simulink model "MQP_RHOME_2025"  (R2024b)
settings: Solver=VariableStepAuto  StartTime=0.0  StopTime=24  RelTol=1e-3  EnableMultiTasking=on
undefined symbols (not defined in the file): DiscIntNeverNeededParam, Ion, Lithium
libraries: spsSeriesRLCBranchLib x11, simulink x11, powerlib_extras x11, spsVoltageMeasurementLib x10, spsGroundLib x4, dspmathops x3, spsUniversalBridgeLib x3, spsMeanLib x3, slpidlib x3, spsCurrentMeasurementLib x2, spsMosfetLib x2, spsThreePhaseParallelRLCBranchLib x2
(part 1 of 3)
settings Model: SimulationMode=accelerator  Creator=yaju  LastModifiedBy=thomasrua
settings SolverCC: AlgebraicLoopSolver=TrustRegion
settings DataIOCC: ReturnWorkspaceOutputs=off
settings OptimizationCC: LifeSpan=inf
settings DebuggingCC: UnconnectedInputMsg=warning  UnconnectedOutputMsg=warning  UnconnectedLineMsg=warning  SFUnexpectedBacktrackingDiag=warning  SFNoUnconditionalDefaultTransitionDiag=warning  SFExecutionAtInitializationDiag=none  ArithmeticOperatorsInVariantConditions=warning
settings ModelReferenceCC: EnableRefExpFcnMdlSchedulingChecks=on
settings SFSimCC: SimUseLocalCustomCode=off  CustomCodeUndefinedFunction=UseInterfaceOnly
settings RTWCC: RTWUseLocalCustomCode=off  GPUComputeCapability=3.5
settings CodeAppCC: StateflowObjectComments=on
settings GRTTargetCC: TargetLangStandard=C89/C90 (ANSI)
settings ConfigComp: CovMetricSettings=dw  CovSaveCumulativeToWorkspaceVar=on  CovSaveSingleToWorkspaceVar=on  CovExternalEMLEnable=off
settings SimscapeCC: SimscapeNormalizeSystem=off

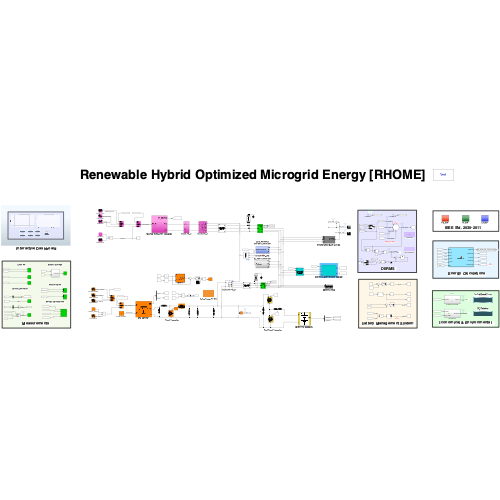
[thumbnail: Simulink's stored preview of the top-level diagram]
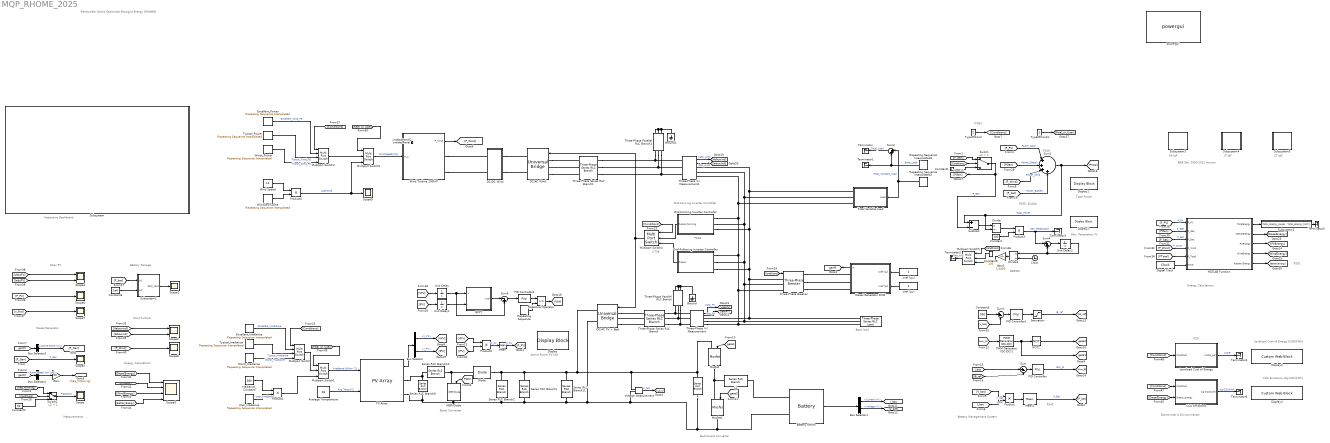
== system MQP_RHOME_2025 ==
  note: Levelized Cost of Energy
      | [USD/kWh]
  note: IT20
  note: PS48
  note: PS49
  note: PS51
  note: PS55: SCADA
  note: PS42
  note: CT39
  note: ITN01
  note: IEEE Std. 2030-2011 Axioms
  note: Economical & Environmental
  note: Grid-Forming
      | Inverter Controller
  note: Measurements
  note: DERMS
  note: Base load
  note: Battery Management System
  note: Buck/boost Converter
  note: Renewable Hybrid Optimized Microgrid Energy [RHOME]
  note: Active Power PV [W]
  note: Interactive Dashboard
  note: Boost Converter
  note: Energy Calculations
  note: Total Power
  note: Ren. Penetration %
  note: Diesel Generator
  note: Solar PV
  note: Battery Storage
  note: Wind Turbine
  note: Energy Calculations
  note: PS-IAP
  note: CT-IAP
  note: IT-IAP
  note: CO2 Emissions
      | [Kg-CO2/kWh]
  " " : spsThreePhaseSeriesRLCLoadLib/Three-Phase Series RLC Load  LConnTagsString=A|B|C  Configuration=Y (grounded)  NominalVoltage=400  Vabc=[1e3 1e3 1e3]  Vabcp=[1e3 1e3 1e3]  NominalFrequency=50  UnbalancedPower=off  ActivePower=83e3  InductivePower=5e3  CapacitivePower=5e3  Pabc=[10e3 9e3 11e3]  QLabc=[100 90 110]  QCabc=[100 90 110]  Pabcp=[10e3 9e3 11e3]  QLabcp=[100 90 110]  QCabcp=[100 90 110]  Measurements=Branch voltages and currents  LoadType=constant PQ
  "      R" : spsSeriesRLCBranchLib/Series RLC Branch  LConnTagsString=__new0  RConnTagsString=__new0  BranchType=RC  Resistance=1e-4  Inductance=1000e-6  SetiL0=off  InitialCurrent=0  Capacitance=210e-6  Setx0=off  InitialVoltage=0  Measurements=None
  "Average Temperature " : Constant  Value=28
  "Battery 6MWh " : spsBatteryLib/Battery  BatType=Lithium-Ion  NomV=230  NomQ=26087  SOC=50  Batt_Tr=1  PresetModel=on  MaxQ=26087  MinV=172.5  FullV=267.717  Dis_rate=11342.1739  R=8.8167e-05  Normal_OP=23591.7217  expZone="[248.48875      1281.6657]"
      settings: LibrarySourceBlock=electricdrivelib/Extra Sources/Battery
  Bus Selector : BusSelector  OutputSignals=V_PV,I_PV
  Bus Selector1 : BusSelector  OutputSignals=Current (A),Voltage (V)
  Bus Selector3 : BusSelector  OutputSignals=Active Power (W)
  Bus Selector4 : BusSelector  OutputSignals="Rotor speed  wm  (pu)"
  CO2 Emissions : Subsystem
  Clock : Clock
  Constant : Constant  Value=100
  Constant1 : Constant  Value=0
  Constant2 : Constant  Value=50
  Constant3 : Constant  Value=550
  Constant4 : Constant  Value=1e6
  Constant5 : Constant  Value=100
  DC/AC PV + Batt : spsUniversalBridgeLib/Universal Bridge  Arms=3  SnubberResistance=1e5  SnubberCapacitance=inf  Device=MOSFET / Diodes  Ron=1e-3  Lon=0  ForwardVoltages="[  0  0  ]"  ForwardVoltage=0  GTOparameters=[ 10e-6 , 20e-6 ]  IGBTparameters=[ 1e-6 , 2e-6 ]  Measurements=None  Measurements_2=None  converterType=Rectifier
  DC/AC Wind : spsUniversalBridgeLib/Universal Bridge  Arms=3  SnubberResistance=1e5  SnubberCapacitance=inf  Device=MOSFET / Diodes  Ron=1e-3  Lon=0  ForwardVoltages="[  0  0  ]"  ForwardVoltage=0  GTOparameters=[ 10e-6 , 20e-6 ]  IGBTparameters=[ 1e-6 , 2e-6 ]  Measurements=None  Measurements_2=None  converterType=Rectifier
  DC/DC Wind : Subsystem
  Diesel Generator 1MW : Subsystem  mask(Diesel Generator (Simple)){Pn=1e6, Vn=285, Fn=50, genType=PQ, PQ0=[0.05 0]}
      mask prompts: Pn "Generator Rated Power [W]"; Vn "Rated Voltage [V]"; Fn "Rated Frequency [Hz]"; genType "Load Flow Type"; PQ0 "Initial Power, [P0 Q0] [pu]"
      mask help:
      | The Diesel Generator block contains a synchronous generator, diesel governor and excitation system to represent the dynamics of a Genset. To inspect the model, look under the block mask (Ctrl + u).
      |
      | The inputs to the basic Diesel generator block are the desired speed reference (in pu) and the desired voltage reference (in pu). The output measurements are contained in a Simulink bus, which can be selected by using the Bus Selector block.
      |
      | Note: The initial generator power must be specified for use for Load Flow analysis.
      mask init:
      | % Extract Initial Active/Reactive Power
      | P0 = PQ0(1);
      | Q0 = PQ0(2);
      | 
      | % Select Load Flow Type
      | genBlock = [gcb '/Synchronous Machine'];
      | currentVals = get_param(genBlock,'MaskValues');
      | currentVals{31} = genType;
      | set_param(genBlock,'MaskValues',currentVals);
      | 
      | % Disable Option if Swing Generator Selected
      | currentEnables = get_param(gcb,'MaskEnables');
      | if strcmp(genType,'swing')
      |     currentEnables{5} = 'off';
      | else
      |     currentEnables{5} = 'on';
      | end
      | set_param(gcb,'MaskEnables',currentEnables);
      mask TypeOptions genType: swing | PQ | PV
  Digital Clock : DigitalClock
  Diode : spsDiodeLib/Diode  Ron=0.001  Lon=0  Vf=0.8  IC=0  UseSnubber=0  Rs=500  Cs=250e-9  Measurements=off
  Display : DisplayBlock  LabelPosition=Hide  Format=Integer  Transparency=1
  Display1 : DisplayBlock  LabelPosition=Hide  Format=Integer  Transparency=1
  Display2 : DisplayBlock  LabelPosition=Hide  Format=Integer  Transparency=1
  Display3 : CustomWebBlock  LabelPosition=Hide  ShowInitialText=on  Configuration="{\"components\":[{\"name\":\"DisplayComponent\",\"settings\":{\"bold\":false,\"font\":\"DSEG7 Classic\",\"fontColor\":[255,255,200],\"fontSize\":\"14\",\"format\":\"short\",\"formatString\":\"%d\",\"italic\":false,\"position\":[0,0,1,1],\"underline\":false}},{\"name\":\"BackgroundImageComponent\",\"settings\":{\"image\":{\"size\":[300,80],\"src\":\"data:image\\/svg+xml;base64,PHN2ZyBpZD0iZnJhbWUiIHhtbG5zPSJodHRwOi8vd3d3LnczLm9yZy8yMDAwL3N2ZyIgeG1sbnM6eGxpbms9Imh0dHA6Ly93d3cudzMub3JnLzE5OTkveGxpbmsiIHZpZXdCb3g9IjAgMCAzODAgMTAxIj48ZGVmcz48c3R5bGU+LmNscy0xe2ZpbGw6IzAwMmI0Mjt9LmNscy0ye2ZpbGw6IzQyNzA4Mjt9LmNscy0ze2ZpbGw6dXJsKCNyYWRpYWwtZ3JhZGllbnQpO308L3N0eWxlPjxyYWRpYWxHcmFkaWVudCBpZD0icmFkaWFsLWdyYWRpZW50IiBjeD0iMTkwIiBjeT0iNTAuNSIgcj0iMjY5LjIxIiBncmFkaWVudFVuaXRzPSJ1c2VyU3BhY2VPblVzZSI+PHN0b3Agb2Zmc2V0PSIwLjAxIiBzdG9wLWNvbG9yPSIjM2U0ZjU4Ii8+PHN0b3Agb2Zmc2V0PSIwLjA2IiBzdG9wLWNvbG9yPSIjNDQ1NzYxIi8+PHN0b3Agb2Zmc2V0PSIwLjE1IiBzdG9wLWNvbG9yPSIjNTU2YTc2Ii8+PHN0b3Agb2Zmc2V0PSIwLjI1IiBzdG9wLWNvbG9yPSIjNmQ4ODk1Ii8+PHN0b3Agb2Zmc2V0PSIwLjM4IiBzdG9wLWNvbG9yPSIjOGZiMmMzIi8+PHN0b3Agb2Zmc2V0PSIwLjUyIiBzdG9wLWNvbG9yPSIjYjZlNGZhIi8+PHN0b3Agb2Zmc2V0PSIxIiBzdG9wLWNvbG9yPSIjMTU0NjU3Ii8+PC9yYWRpYWxHcmFkaWVudD48L2RlZnM+PGcgaWQ9IkxheWVyXzIiIGRhdGEtbmFtZT0iTGF5ZXIgMiI+PGcgaWQ9IkxheWVyXzEtMiIgZGF0YS1uYW1lPSJMYXllciAxLTIiPjxyZWN0IGlkPSJyZWN0MTAzNiIgY2xhc3M9ImNscy0xIiB4PSIxMSIgeT0iMTEiIHdpZHRoPSIzNTgiIGhlaWdodD0iNzkiLz48cGF0aCBpZD0icGF0aDEwMzgiIGNsYXNzPSJjbHMtMiIgZD0iTTgsOFY5M0gzNzJWOFpNMzY5LDkwSDExVjExSDM2OVoiLz48cGF0aCBpZD0icGF0aDEwNDAiIGNsYXNzPSJjbHMtMyIgZD0iTTAsMFYxMDFIMzgwVjBaTTM3Miw5M0g4VjhIMzcyWiIvPjwvZz48L2c+PC9zdmc+\",\"srcOrientation\":\"Right\"},\"position\":[0,0,1,1],\"scaleMode\":\"0\"}},{\"name\":\"ForegroundImageComponent\",\"settings\":{\"angle\":0,\"image\":{\"size\":[0,0],\"src\":\"default\"},\"isForeground\":1,\"position\":[0,0,1,1],\"scaleMode\":\"0\"}}],\"settings\":{\"BindingType\":\"signal\",\"aspectRatio\":1.032258064516129,\"backgroundColor\":[0,0,0,\"1\"],\"backgroundOffset\":0.14,\"backgroundOpacity\":1,\"fixedAspectRatio\":\"on\",\"showBackgroundColor\":false,\"value\":0,\"version\":\"R2023b\"},\"type\":\"Display\"}"
  Display4 : CustomWebBlock  LabelPosition=Hide  ShowInitialText=on  Configuration="{\"components\":[{\"name\":\"DisplayComponent\",\"settings\":{\"bold\":false,\"font\":\"DSEG7 Classic\",\"fontColor\":[255,255,200],\"fontSize\":\"14\",\"format\":\"short\",\"formatString\":\"%d\",\"italic\":false,\"position\":[0,0,1,1],\"underline\":false}},{\"name\":\"BackgroundImageComponent\",\"settings\":{\"image\":{\"size\":[300,80],\"src\":\"data:image\\/svg+xml;base64,PHN2ZyBpZD0iZnJhbWUiIHhtbG5zPSJodHRwOi8vd3d3LnczLm9yZy8yMDAwL3N2ZyIgeG1sbnM6eGxpbms9Imh0dHA6Ly93d3cudzMub3JnLzE5OTkveGxpbmsiIHZpZXdCb3g9IjAgMCAzODAgMTAxIj48ZGVmcz48c3R5bGU+LmNscy0xe2ZpbGw6IzAwMmI0Mjt9LmNscy0ye2ZpbGw6IzQyNzA4Mjt9LmNscy0ze2ZpbGw6dXJsKCNyYWRpYWwtZ3JhZGllbnQpO308L3N0eWxlPjxyYWRpYWxHcmFkaWVudCBpZD0icmFkaWFsLWdyYWRpZW50IiBjeD0iMTkwIiBjeT0iNTAuNSIgcj0iMjY5LjIxIiBncmFkaWVudFVuaXRzPSJ1c2VyU3BhY2VPblVzZSI+PHN0b3Agb2Zmc2V0PSIwLjAxIiBzdG9wLWNvbG9yPSIjM2U0ZjU4Ii8+PHN0b3Agb2Zmc2V0PSIwLjA2IiBzdG9wLWNvbG9yPSIjNDQ1NzYxIi8+PHN0b3Agb2Zmc2V0PSIwLjE1IiBzdG9wLWNvbG9yPSIjNTU2YTc2Ii8+PHN0b3Agb2Zmc2V0PSIwLjI1IiBzdG9wLWNvbG9yPSIjNmQ4ODk1Ii8+PHN0b3Agb2Zmc2V0PSIwLjM4IiBzdG9wLWNvbG9yPSIjOGZiMmMzIi8+PHN0b3Agb2Zmc2V0PSIwLjUyIiBzdG9wLWNvbG9yPSIjYjZlNGZhIi8+PHN0b3Agb2Zmc2V0PSIxIiBzdG9wLWNvbG9yPSIjMTU0NjU3Ii8+PC9yYWRpYWxHcmFkaWVudD48L2RlZnM+PGcgaWQ9IkxheWVyXzIiIGRhdGEtbmFtZT0iTGF5ZXIgMiI+PGcgaWQ9IkxheWVyXzEtMiIgZGF0YS1uYW1lPSJMYXllciAxLTIiPjxyZWN0IGlkPSJyZWN0MTAzNiIgY2xhc3M9ImNscy0xIiB4PSIxMSIgeT0iMTEiIHdpZHRoPSIzNTgiIGhlaWdodD0iNzkiLz48cGF0aCBpZD0icGF0aDEwMzgiIGNsYXNzPSJjbHMtMiIgZD0iTTgsOFY5M0gzNzJWOFpNMzY5LDkwSDExVjExSDM2OVoiLz48cGF0aCBpZD0icGF0aDEwNDAiIGNsYXNzPSJjbHMtMyIgZD0iTTAsMFYxMDFIMzgwVjBaTTM3Miw5M0g4VjhIMzcyWiIvPjwvZz48L2c+PC9zdmc+\",\"srcOrientation\":\"Right\"},\"position\":[0,0,1,1],\"scaleMode\":\"0\"}},{\"name\":\"ForegroundImageComponent\",\"settings\":{\"angle\":0,\"image\":{\"size\":[0,0],\"src\":\"default\"},\"isForeground\":1,\"position\":[0,0,1,1],\"scaleMode\":\"0\"}}],\"settings\":{\"BindingType\":\"signal\",\"aspectRatio\":1.032258064516129,\"backgroundColor\":[0,0,0,\"1\"],\"backgroundOffset\":0.14,\"backgroundOpacity\":1,\"fixedAspectRatio\":\"on\",\"showBackgroundColor\":false,\"value\":0,\"version\":\"R2023b\"},\"type\":\"Display\"}"
  Divide : Product  Inputs=*/
  Divide1 : Product  Inputs=*/
  Excellent_Irradiance : simulink/Sources/Repeating Sequence Interpolated  OutValues=[1 2 3 4 6 15 25 44.75 266.65 518.2 750.55 939.2 1029.35 1044.75 955.25 818.67 608.55 354.08 102.43 60 40 22 5 2]  TimeValues=[0 1 2 3 4 5 6 7 8 9 10 11 12 13 14 15 16 17 18 19 20 21 22 23]  LookUpMeth=Interpolation-Use End Values  tsamp=1e-6  OutMin=[]  OutMax=[]  OutDataTypeStr=double  OutputDataTypeScalingMode=double  OutDataType=fixdt(0,8)  OutScaling=2^-10
  Excellent_Power : simulink/Sources/Repeating Sequence Interpolated  OutValues=[10 9 9 9 8 8 7 6 9 10 9 8 8 7 7 7 8 9 10 10 9 8 7 6]  TimeValues=[0 1 2 3 4 5 6 7 8 9 10 11 12 13 14 15 16 17 18 19 20 21 22 23]  LookUpMeth=Interpolation-Use End Values  tsamp=1e-6  OutMin=[]  OutMax=[]  OutDataTypeStr=double  OutputDataTypeScalingMode=double  OutDataType=fixdt(0,8)  OutScaling=2^-10
  Gain : Gain  Gain=50
  Gain1 : Gain  Gain=1/1000
  Grid-Following Inverter Controller : Subsystem
  Grid-Forming Inverter Controller : Subsystem
  Ground : spsGroundLib/Ground  LConnTagsString=a
  Ground1 : spsGroundLib/Ground  LConnTagsString=a
  IGBT/Diode : spsIGBTDiodeLib/IGBT//Diode  Ron=1e-3  Rs=1e5  Cs=inf  Measurements=off
  Irradiance_Constant : Constant  Value=380
  L1 : spsSeriesRLCBranchLib/Series RLC Branch  LConnTagsString=__new0  RConnTagsString=__new0  BranchType=RL  Resistance=1e-4  Inductance=6.4e-3  SetiL0=off  InitialCurrent=0  Capacitance=1e-6  Setx0=off  InitialVoltage=0  Measurements=None
  Levelized Cost of Energy : Subsystem
  MATLAB Function : MATLAB Function  TreatAsAtomicUnit=on
  MPPT : MATLAB Function  TreatAsAtomicUnit=on
  Mean : spsMeanLib/Mean  Freq=50  Vinit=0  Ts=1e-6
  Mean1 : spsMeanLib/Mean  Freq=50  Vinit=0  Ts=1e-6
  Mosfet : spsMosfetLib/Mosfet  Ron=0.1  Lon=0  Rd=0.01  Vfd=0  IC=0  Rs=1e5  Cs=inf  Measurements=off
  Mosfet1 : spsMosfetLib/Mosfet  Ron=0.1  Lon=0  Rd=0.01  Vfd=0  IC=0  Rs=1e5  Cs=inf  Measurements=off
  Multiport Switch : MultiPortSwitch  SaturateOnIntegerOverflow=off  InputSameDT=off
  Multiport Switch{1,3..5} (4 alike) : MultiPortSwitch  Inputs=2  SaturateOnIntegerOverflow=off  InputSameDT=off
      Multiport Switch4 mask Display: image('CT39.jpg');
  Multiport Switch2 : MultiPortSwitch  SaturateOnIntegerOverflow=off  InputSameDT=off
  NOT2 : Logic  Operator=NOT  AllPortsSameDT=off  OutDataTypeStr=boolean
  PID Controller : slpidlib/PID Controller  Controller=PI  Form=Parallel  TimeDomain=Discrete-time  UseExternalTs=off  SampleTime=50e-6  IntegratorMethod=Forward Euler  FilterMethod=Forward Euler  ControllerParametersSource=internal  P=0.01  I=5  UseKiTs=off  D=0  UseExternalDerivativeSource=off  N=100  UseFilter=on  TunerSelectOption=Transfer Function Based (PID Tuner App)  InitialConditionSource=internal  InitialConditionForIntegrator=0  InitialConditionForFilter=0  DifferentiatorICPrevScaledInput=0  ExternalReset=none  TrackingMode=off  Kt=1  LimitOutput=on  SatLimitsSource=internal  UpperSaturationLimit=0.95  LowerSaturationLimit=0  LinearizeAsGain=on  AntiWindupMode=none  Kb=1  LimitIntegrator=off  UpperIntegratorSaturationLimit=inf  LowerIntegratorSaturationLimit=-inf  POutMin=[]  POutMax=[]  IOutMin=[]  IOutMax=[]  DOutMin=[]  DOutMax=[]  NOutMin=[]  NOutMax=[]  SumOutMin=[]  SumOutMax=[]  SaturationOutMin=[]  SaturationOutMax=[]  PParamMin=[]  PParamMax=[]  IParamMin=[]  IParamMax=[]  DParamMin=[]  DParamMax=[]  NParamMin=[]  NParamMax=[]  KbParamMin=[]  KbParamMax=[]  KtParamMin=[]  KtParamMax=[]  KbOutMin=[]  KbOutMax=[]  KtOutMin=[]  KtOutMax=[]  IntegratorOutMin=[]  IntegratorOutMax=[]  FilterOutMin=[]  FilterOutMax=[]  SumI1OutMin=[]  SumI1OutMax=[]  SumI2OutMin=[]  SumI2OutMax=[]  SumI3OutMin=[]  SumI3OutMax=[]  SumI4OutMin=[]  SumI4OutMax=[]  SumDOutMin=[]  SumDOutMax=[]  DifferentiatorOutMin=[]  DifferentiatorOutMax=[]  FilterDiffOutCoefMin=[]  FilterDiffOutCoefMax=[]  ReciprocalOutMin=[]  ReciprocalOutMax=[]  SumDenOutMin=[]  SumDenOutMax=[]  SumNumOutMin=[]  SumNumOutMax=[]  DivideOutMin=[]  DivideOutMax=[]  UdiffTsProdOutMin=[]  UdiffTsProdOutMax=[]  NTsProdOutMin=[]  NTsProdOutMax=[]  UintegralTsProdOutMin=[]  UintegralTsProdOutMax=[]  UngainTsProdOutMin=[]  UngainTsProdOutMax=[]  ClampingZeroOutDataTypeStr=Inherit: Inherit via back propagation  ClampingZeroOutMin=[]  ClampingZeroOutMax=[]  FilterDenConstantOutDataTypeStr=Inherit: Inherit via back propagation  FilterDenConstantOutMin=[]  FilterDenConstantOutMax=[]  PCopyOutDataTypeStr=Inherit: Inherit via back propagation  PCopyOutMin=[]  PCopyOutMax=[]  NCopyOutDataTypeStr=Inherit: Inherit via back propagation  NCopyOutMin=[]  NCopyOutMax=[]  IntegratorContinuousStateAttributes=''  IntegratorStateMustResolveToSignalObject=off  IntegratorRTWStateStorageClass=Auto  FilterContinuousStateAttributes=''  FilterStateMustResolveToSignalObject=off  FilterRTWStateStorageClass=Auto  ParallelPVariant=InternalParameters  IdealPVariant=Disabled  IVariant=InternalParameters  DVariant=Disabled  IntegratorVariant=Discrete  SatVariant=Enabled  AWVariant=Passthrough  PCopyVariant=Disabled  TRVariant=Disabled  FdbkBlocksVariant=Forward  IdealPFdbkVariant=Disabled  SatFdbkVariant=Disabled  DerivativeFilterVariant=Disabled  NVariant=Disabled  NCopyVariant=Disabled_SignalSpec  FilterICVariant=Disabled  IntegratorICVariant=InternalICs  ExternalResetVariant=Disabled  TRSumVariant=Passthrough  SumFdbkVariant=Disabled  SumVariant=Sum_PI  TsampFilterVariant=InternalTs  TsampNgainVariant=Passthrough  TsampIntegralVariant=Disabled_SignalSpec  ExternalSaturationOutDataTypeStr=Inherit: Same as second input  DerivativeSourceVariant=Disabled  PreIntVariant=InternalPreInt
  PID Controller1 : slpidlib/PID Controller  Controller=PI  Form=Parallel  TimeDomain=Discrete-time  UseExternalTs=off  SampleTime=500e-6  IntegratorMethod=Forward Euler  FilterMethod=Forward Euler  ControllerParametersSource=internal  P=0.5  I=5  UseKiTs=off  D=0  UseExternalDerivativeSource=off  N=100  UseFilter=on  TunerSelectOption=Transfer Function Based (PID Tuner App)  InitialConditionSource=internal  InitialConditionForIntegrator=0  InitialConditionForFilter=0  DifferentiatorICPrevScaledInput=0  ExternalReset=none  TrackingMode=off  Kt=1  LimitOutput=on  SatLimitsSource=internal  UpperSaturationLimit=1  LowerSaturationLimit=-1  LinearizeAsGain=on  AntiWindupMode=back-calculation  Kb=1  LimitIntegrator=on  UpperIntegratorSaturationLimit=1  LowerIntegratorSaturationLimit=-1  POutMin=[]  POutMax=[]  IOutMin=[]  IOutMax=[]  DOutMin=[]  DOutMax=[]  NOutMin=[]  NOutMax=[]  SumOutMin=[]  SumOutMax=[]  SaturationOutMin=[]  SaturationOutMax=[]  PParamMin=[]  PParamMax=[]  IParamMin=[]  IParamMax=[]  DParamMin=[]  DParamMax=[]  NParamMin=[]  NParamMax=[]  KbParamMin=[]  KbParamMax=[]  KtParamMin=[]  KtParamMax=[]  KbOutMin=[]  KbOutMax=[]  KtOutMin=[]  KtOutMax=[]  IntegratorOutMin=[]  IntegratorOutMax=[]  FilterOutMin=[]  FilterOutMax=[]  SumI1OutMin=[]  SumI1OutMax=[]  SumI2OutMin=[]  SumI2OutMax=[]  SumI3OutMin=[]  SumI3OutMax=[]  SumI4OutMin=[]  SumI4OutMax=[]  SumDOutMin=[]  SumDOutMax=[]  DifferentiatorOutMin=[]  DifferentiatorOutMax=[]  FilterDiffOutCoefMin=[]  FilterDiffOutCoefMax=[]  ReciprocalOutMin=[]  ReciprocalOutMax=[]  SumDenOutMin=[]  SumDenOutMax=[]  SumNumOutMin=[]  SumNumOutMax=[]  DivideOutMin=[]  DivideOutMax=[]  UdiffTsProdOutMin=[]  UdiffTsProdOutMax=[]  NTsProdOutMin=[]  NTsProdOutMax=[]  UintegralTsProdOutMin=[]  UintegralTsProdOutMax=[]  UngainTsProdOutMin=[]  UngainTsProdOutMax=[]  ClampingZeroOutDataTypeStr=Inherit: Inherit via back propagation  ClampingZeroOutMin=[]  ClampingZeroOutMax=[]  FilterDenConstantOutDataTypeStr=Inherit: Inherit via back propagation  FilterDenConstantOutMin=[]  FilterDenConstantOutMax=[]  PCopyOutDataTypeStr=Inherit: Inherit via back propagation  PCopyOutMin=[]  PCopyOutMax=[]  NCopyOutDataTypeStr=Inherit: Inherit via back propagation  NCopyOutMin=[]  NCopyOutMax=[]  IntegratorContinuousStateAttributes=''  IntegratorStateMustResolveToSignalObject=off  IntegratorRTWStateStorageClass=Auto  FilterContinuousStateAttributes=''  FilterStateMustResolveToSignalObject=off  FilterRTWStateStorageClass=Auto  ParallelPVariant=InternalParameters  IdealPVariant=Disabled  IVariant=InternalParameters  DVariant=Disabled  IntegratorVariant=Discrete  SatVariant=Enabled  AWVariant=BackCalculation  PCopyVariant=Disabled  TRVariant=Disabled  FdbkBlocksVariant=Forward  IdealPFdbkVariant=Disabled  SatFdbkVariant=Disabled  DerivativeFilterVariant=Disabled  NVariant=Disabled  NCopyVariant=Disabled_SignalSpec  FilterICVariant=Disabled  IntegratorICVariant=InternalICs  ExternalResetVariant=Disabled  TRSumVariant=Passthrough  SumFdbkVariant=Disabled  SumVariant=Sum_PI  TsampFilterVariant=InternalTs  TsampNgainVariant=Passthrough  TsampIntegralVariant=Disabled_SignalSpec  ExternalSaturationOutDataTypeStr=Inherit: Same as second input  DerivativeSourceVariant=Disabled  PreIntVariant=InternalPreInt
  PID Controller4 : slpidlib/PID Controller  Controller=PI  Form=Parallel  TimeDomain=Continuous-time  UseExternalTs=off  SampleTime=-1  IntegratorMethod=Forward Euler  FilterMethod=Forward Euler  ControllerParametersSource=internal  P=0.05  I=0.0001  UseKiTs=off  D=0  UseExternalDerivativeSource=off  N=100  UseFilter=on  TunerSelectOption=Transfer Function Based (PID Tuner App)  InitialConditionSource=internal  InitialConditionForIntegrator=0  InitialConditionForFilter=0  DifferentiatorICPrevScaledInput=0  ExternalReset=none  TrackingMode=off  Kt=1  LimitOutput=on  SatLimitsSource=internal  UpperSaturationLimit=0.95  LowerSaturationLimit=0  LinearizeAsGain=on  AntiWindupMode=none  Kb=1  LimitIntegrator=off  UpperIntegratorSaturationLimit=inf  LowerIntegratorSaturationLimit=-inf  POutMin=[]  POutMax=[]  IOutMin=[]  IOutMax=[]  DOutMin=[]  DOutMax=[]  NOutMin=[]  NOutMax=[]  SumOutMin=[]  SumOutMax=[]  SaturationOutMin=[]  SaturationOutMax=[]  PParamMin=[]  PParamMax=[]  IParamMin=[]  IParamMax=[]  DParamMin=[]  DParamMax=[]  NParamMin=[]  NParamMax=[]  KbParamMin=[]  KbParamMax=[]  KtParamMin=[]  KtParamMax=[]  KbOutMin=[]  KbOutMax=[]  KtOutMin=[]  KtOutMax=[]  IntegratorOutMin=[]  IntegratorOutMax=[]  FilterOutMin=[]  FilterOutMax=[]  SumI1OutMin=[]  SumI1OutMax=[]  SumI2OutMin=[]  SumI2OutMax=[]  SumI3OutMin=[]  SumI3OutMax=[]  SumI4OutMin=[]  SumI4OutMax=[]  SumDOutMin=[]  SumDOutMax=[]  DifferentiatorOutMin=[]  DifferentiatorOutMax=[]  FilterDiffOutCoefMin=[]  FilterDiffOutCoefMax=[]  ReciprocalOutMin=[]  ReciprocalOutMax=[]  SumDenOutMin=[]  SumDenOutMax=[]  SumNumOutMin=[]  SumNumOutMax=[]  DivideOutMin=[]  DivideOutMax=[]  UdiffTsProdOutMin=[]  UdiffTsProdOutMax=[]  NTsProdOutMin=[]  NTsProdOutMax=[]  UintegralTsProdOutMin=[]  UintegralTsProdOutMax=[]  UngainTsProdOutMin=[]  UngainTsProdOutMax=[]  ClampingZeroOutDataTypeStr=Inherit: Inherit via back propagation  ClampingZeroOutMin=[]  ClampingZeroOutMax=[]  FilterDenConstantOutDataTypeStr=Inherit: Inherit via back propagation  FilterDenConstantOutMin=[]  FilterDenConstantOutMax=[]  PCopyOutDataTypeStr=Inherit: Inherit via back propagation  PCopyOutMin=[]  PCopyOutMax=[]  NCopyOutDataTypeStr=Inherit: Inherit via back propagation  NCopyOutMin=[]  NCopyOutMax=[]  IntegratorContinuousStateAttributes=''  IntegratorStateMustResolveToSignalObject=off  IntegratorRTWStateStorageClass=Auto  FilterContinuousStateAttributes=''  FilterStateMustResolveToSignalObject=off  FilterRTWStateStorageClass=Auto  ParallelPVariant=InternalParameters  IdealPVariant=Disabled  IVariant=InternalParameters  DVariant=Disabled  IntegratorVariant=Continuous  SatVariant=Enabled  AWVariant=Passthrough  PCopyVariant=Disabled  TRVariant=Disabled  FdbkBlocksVariant=Forward  IdealPFdbkVariant=Disabled  SatFdbkVariant=Disabled  DerivativeFilterVariant=Disabled  NVariant=Disabled  NCopyVariant=Disabled_SignalSpec  FilterICVariant=Disabled  IntegratorICVariant=InternalICs  ExternalResetVariant=Disabled  TRSumVariant=Passthrough  SumFdbkVariant=Disabled  SumVariant=Sum_PI  TsampFilterVariant=InternalTs  TsampNgainVariant=Passthrough  TsampIntegralVariant=Disabled_SignalSpec  ExternalSaturationOutDataTypeStr=Inherit: Same as second input  DerivativeSourceVariant=Disabled  PreIntVariant=InternalPreInt
  "PV Array " : spsPVArrayLib/PV Array  Npar=660  Nser=10  PlotType=array @ 25 deg.C & specified irradiances  S_vec="[ 1000  900  800 ]"  Temp_C_vec="[ 45 25  ]"  ModuleName=User-defined  PlotWhenSelected=off  Pm=213.15  Ncell=60  Voc=36.3  Isc=7.84  Vm=29  Im=7.35  beta_Voc_pc=-0.36099  alpha_Isc_pc=0.102  beta_Voc=-0.13104  alpha_Isc=0.0079968  IL=7.8654  I0=2.9273e-10  nI=0.98119  Rsh=313.0553  Rs=0.39381  RobustModel=off  RobustCellTemperature=313.3991  BAL=on  Tc=1e-6  Tfilter=5e-5
  PWM Generator (DC-DC)1 : spsPWMGeneratorDCDCLib/PWM Generator (DC-DC)  Fsw=10000  Ts=1e-6
  Product{,1..4} (5 alike) : Product
  Relational Operator : RelationalOperator  OutDataTypeStr=boolean  RndMeth=Simplest  InputSameDT=off
  Repeating Sequence : simulink/Sources/Repeating Sequence  rep_seq_t=[0 0.0001 0.0002]  rep_seq_y=[-1 1 -1]
  Repeating Sequence Interpolated2 : simulink/Sources/Repeating Sequence Interpolated  OutValues=[0 0 0 0 13410 115850 141460 115850 56100 64630 107320 124390 226830 115860 56100 39000 47560 192680 538780 448780 209760 73120 0 0]  TimeValues=[0 1 2 3 4 5 6 7 8 9 10 11 12 13 14 15 16 17 18 19 20 21 22 23]  LookUpMeth=Interpolation-Use End Values  tsamp=1e-6  OutMin=[]  OutMax=[]  OutDataTypeStr=double  OutputDataTypeScalingMode=double  OutDataType=fixdt(0,8)  OutScaling=2^-10
  Repeating Sequence Interpolated4 : simulink/Sources/Repeating Sequence Interpolated  OutValues=[200000 200000 200000 200000 200000 200000 200000 200000 200000 200000 200000 200000 200000 200000 200000 200000 200000 200000 200000 200000 200000 200000 200000 200000]  TimeValues=[0 1 2 3 4 5 6 7 8 9 10 11 12 13 14 15 16 17 18 19 20 21 22 23]  LookUpMeth=Interpolation-Use End Values  tsamp=1e-6  OutMin=[]  OutMax=[]  OutDataTypeStr=double  OutputDataTypeScalingMode=double  OutDataType=fixdt(0,8)  OutScaling=2^-10
  Saturation : Saturate  UpperLimit=1  LowerLimit=-1
  Scope{,1..2,6..9} (7 alike) : Scope
  Scope3 : Scope  NumInputPorts=2
  Scope4 : Scope  NumInputPorts=2
  Scope5 : Scope  NumInputPorts=4
  Series RLC Branch1 : spsSeriesRLCBranchLib/Series RLC Branch  LConnTagsString=__new0  RConnTagsString=__new0  BranchType=R  Resistance=0.23  Inductance=1e-3  SetiL0=off  InitialCurrent=0  Capacitance=3227e-6  Setx0=off  InitialVoltage=0  Measurements=None
  Series RLC Branch10 : spsSeriesRLCBranchLib/Series RLC Branch  LConnTagsString=__new0  RConnTagsString=__new0  BranchType=L  Resistance=1  Inductance=4.133e-3  SetiL0=off  InitialCurrent=0  Capacitance=1e-6  Setx0=off  InitialVoltage=0  Measurements=None
  Series RLC Branch11 : spsSeriesRLCBranchLib/Series RLC Branch  LConnTagsString=__new0  RConnTagsString=__new0  BranchType=RC  Resistance=1e-4  Inductance=1e-3  SetiL0=off  InitialCurrent=0  Capacitance=803.6e-6  Setx0=off  InitialVoltage=0  Measurements=None
  Series RLC Branch2 : spsSeriesRLCBranchLib/Series RLC Branch  LConnTagsString=__new0  RConnTagsString=__new0  BranchType=C  Resistance=1  Inductance=1e-3  SetiL0=off  InitialCurrent=0  Capacitance=0.052682  Setx0=off  InitialVoltage=0  Measurements=None
  Series RLC Branch9 : spsSeriesRLCBranchLib/Series RLC Branch  LConnTagsString=__new0  RConnTagsString=__new0  BranchType=RC  Resistance=1e-3  Inductance=1e-3  SetiL0=off  InitialCurrent=0  Capacitance=1000e-6  Setx0=off  InitialVoltage=0  Measurements=None
  Subsystem : Subsystem
  Subsystem1 : Subsystem
  Subsystem2 : Subsystem
  Subsystem3 : Subsystem
  Subsystem4 : Subsystem
  Subsystem5 : Subsystem
  Subtract : Sum  Inputs=+-
  Sum : Sum  Inputs=|+-
  Sum1 : Sum  Inputs=|+-
  Sum2 : Sum  Inputs=|++++
  Sum3 : Sum  Inputs=|++
  Sum4 : Sum  Inputs=|++
  Sum9 : Sum  Inputs=|-+
  Switch : Switch  Criteria=u2 > Threshold  Threshold=1  SaturateOnIntegerOverflow=off  InputSameDT=off
  Switch1 : Switch  Criteria=u2 > Threshold  Threshold=1  SaturateOnIntegerOverflow=off  InputSameDT=off
  Terminator{,1..6} (7 alike) : Terminator
  Three-Phase Parallel RLC Branch : spsThreePhaseParallelRLCBranchLib/Three-Phase Parallel RLC Branch  LConnTagsString=A|B|C  RConnTagsString=A|B|C  BranchType=C  Resistance=1  Inductance=1e-3  Capacitance=13.5e-5  Measurements=None
  Three-Phase Parallel RLC Branch1 : spsThreePhaseParallelRLCBranchLib/Three-Phase Parallel RLC Branch  LConnTagsString=A|B|C  RConnTagsString=A|B|C  BranchType=C  Resistance=1  Inductance=1e-3  Capacitance=13.5e-5  Measurements=None
  Three-Phase Series RLC Branch : spsThreePhaseSeriesRLCBranchLib/Three-Phase Series RLC Branch  LConnTagsString=A|B|C  RConnTagsString=A|B|C  BranchType=RL  Resistance=2  Inductance=1e-2  Capacitance=15.5e-5  Measurements=None
  Three-Phase Series RLC Branch1 : spsThreePhaseSeriesRLCBranchLib/Three-Phase Series RLC Branch  LConnTagsString=A|B|C  RConnTagsString=A|B|C  BranchType=RL  Resistance=2  Inductance=1e-2  Capacitance=15.5e-5  Measurements=None
  Three-Phase V-I Measurement : spsThreePhaseVIMeasurementLib/Three-Phase V-I Measurement  VoltageMeasurement=phase-to-phase  SetLabelV=off  LabelV=Vabc  Vpu=off  VpuLL=off  CurrentMeasurement=yes  SetLabelI=off  LabelI=Iabc  Ipu=off  Pbase=100e6  Vbase=500e3  OutputType=Complex  PhasorSimulation=off  PSBequivalent=0
  Three-Phase V-I Measurement1 : spsThreePhaseVIMeasurementLib/Three-Phase V-I Measurement  VoltageMeasurement=phase-to-phase  SetLabelV=off  LabelV=Vabc  Vpu=off  VpuLL=off  CurrentMeasurement=yes  SetLabelI=off  LabelI=Iabc  Ipu=off  Pbase=100e6  Vbase=500e3  OutputType=Complex  PhasorSimulation=off  PSBequivalent=0
  Three-Phase Breaker : spsThreePhaseBreakerLib/Three-Phase Breaker  InitialState=closed  SwitchA=on  SwitchB=on  SwitchC=on  SwitchTimes=[1/60 5/60]  External=on  BreakerResistance=0.01  SnubberResistance=1e6  SnubberCapacitance=inf  Measurements=None
  "Total Variable Load " : Subsystem  mask(Variable Load (PQ Model)){Vn=400, Fn=50, PF=1, Load0=50e3}
      mask prompts: Vn "Nominal L-L Voltage [Vrms]"; Fn "Nominal Frequency [Hz]"; PF "Power Factor [0 to 1]"; Load0 "Initial Load [W]"
      mask help:
      | The Variable Load block is a lumped approximation for a distribution feeder. For non-unity power factor loads, the input (active power) is scaled accordingly to generate a desired load.
      |
      | Note: The initial input load must be specified for use for Load Flow analysis.
      mask init:
      | P0 = Load0;
      | Q0 = Load0*sqrt(1/PF-1);
  TypeOfCond : Constant  Value=2
  TypeOfCond1 : Constant
  Typical_Irradiance : simulink/Sources/Repeating Sequence Interpolated  OutValues=[0 0 0 0 2 4 92 246 463 735 871 928 829 691 392 269 118 14 5 2 0 0 0 0]  TimeValues=[0 1 2 3 4 5 6 7 8 9 10 11 12 13 14 15 16 17 18 19 20 21 22 23]  LookUpMeth=Interpolation-Use End Values  tsamp=1e-6  OutMin=[]  OutMax=[]  OutDataTypeStr=double  OutputDataTypeScalingMode=double  OutDataType=fixdt(0,8)  OutScaling=2^-10
  Typical_Power : simulink/Sources/Repeating Sequence Interpolated  OutValues=[6.23 5.48 5.3 5.98 6.48 6.48 6.04 5.16 4.92 4.94 4.92 4.84 4.67 4.51 4.47 4.58 4.71 4.77 4.76 4.79 4.86 4.86 4.87 5.1]  TimeValues=[0 1 2 3 4 5 6 7 8 9 10 11 12 13 14 15 16 17 18 19 20 21 22 23]  LookUpMeth=Interpolation-Use End Values  tsamp=1e-6  OutMin=[]  OutMax=[]  OutDataTypeStr=double  OutputDataTypeScalingMode=double  OutDataType=fixdt(0,8)  OutScaling=2^-10
  Unit Delay : UnitDelay  SampleTime=1e-6  HasFrameUpgradeWarning=on
  Unit Delay1 : UnitDelay  SampleTime=1e-6  HasFrameUpgradeWarning=on
  Unit Delay2 : UnitDelay  SampleTime=1e-3  HasFrameUpgradeWarning=on
  User_Irradiance : simulink/Sources/Repeating Sequence Interpolated  OutValues=[0.002 0.003 0.004 0.004 0.006 0.007 0.057 0.271 0.517 0.711 0.855 0.916 0.912 0.789 0.664 0.461 0.253 0.045 0.015 0.007 0.006 0.004 0.003 0.003]  TimeValues=[0 1 2 3 4 5 6 7 8 9 10 11 12 13 14 15 16 17 18 19 20 21 22 23]  LookUpMeth=Interpolation-Use End Values  tsamp=1e-6  OutMin=[]  OutMax=[]  OutDataTypeStr=double  OutputDataTypeScalingMode=double  OutDataType=fixdt(0,8)  OutScaling=2^-10
  Voltage Measurement : spsVoltageMeasurementLib/Voltage Measurement  PhasorSimulation=off  OutputType=Complex  PSBequivalent=0
  Vref (pu) : Constant
  Wind Speed : Constant  Value=11
  Wind Turbine 100kW : Subsystem
  WindZeroToOne : simulink/Sources/Repeating Sequence Interpolated  OutValues=[1.0 0.9 0.9 0.9 0.8 0.8 0.7 0.6 0.9 1.0 0.9 0.8 0.8 0.7 0.7 0.7 0.8 0.9 1.0 1.0 0.9 0.8 0.7 0.6]  TimeValues=[0 1 2 3 4 5 6 7 8 9 10 11 12 13 14 15 16 17 18 19 20 21 22 23]  LookUpMeth=Interpolation-Use End Values  tsamp=1e-6  OutMin=[]  OutMax=[]  OutDataTypeStr=double  OutputDataTypeScalingMode=double  OutDataType=fixdt(0,8)  OutScaling=2^-10
  Worst_Irradiance : simulink/Sources/Repeating Sequence Interpolated  OutValues=[0 0 0 0 0 0 61 118 113 86 102 76 51 56 70 78 65 17 0 0 0 0 0 0]  TimeValues=[0 1 2 3 4 5 6 7 8 9 10 11 12 13 14 15 16 17 18 19 20 21 22 23]  LookUpMeth=Interpolation-Use End Values  tsamp=1e-6  OutMin=[]  OutMax=[]  OutDataTypeStr=double  OutputDataTypeScalingMode=double  OutDataType=fixdt(0,8)  OutScaling=2^-10
  Worst_Power : simulink/Sources/Repeating Sequence Interpolated  OutValues=[2.3 2.3 2.46 2.86 3.29 3.81 4.07 3.13 2.85 3.84 4.45 4.46 3.92 3.25 2.74 2.7 3.33 5.16 7.56 8.83 8.29 6.93 5.97 5.38]  TimeValues=[0 1 2 3 4 5 6 7 8 9 10 11 12 13 14 15 16 17 18 19 20 21 22 23]  LookUpMeth=Interpolation-Use End Values  tsamp=1e-6  OutMin=[]  OutMax=[]  OutDataTypeStr=double  OutputDataTypeScalingMode=double  OutDataType=fixdt(0,8)  OutScaling=2^-10
  powergui : spspowerguiLib/powergui  Priority=1  SimulationMode=Discrete  SampleTime=1e-6  frequency=60  Iterations=50  frequencyindice=0  Pbase=100e6  ErrMax=1e-4  UnitsV=kV  UnitsW=MW  buscounter=0  FunctionMessages=off  echomessages=off  EnableUseOfTLC=off  CurrentSourceSwitches=off  DisableSnubberDevices=off  DisableRonSwitches=off  DisableVfSwitches=off  DisplayEquations=off  AutomaticDiscreteSolvers=off  SolverType=Tustin/Backward Euler (TBE)  Interpol=off  ExternalGateDelay=off  methode=off  Ts=100  x0status=blocks  SPID=off  SwTol=0  HookPort=off  NonlinearTolerance=1e-4  nMaxIteration=100  ContinueOnMaxIteration=off  RestoreLinks=warning  ResistiveCurrentMeasurement=off  Frange=[0:2:500]  Ylog=off  Xlog=on  ShowGrid=off  save=off  variable=ZData  structure=gv1  ZoomFFT=off  StartTime=0.0  cycles=3  DisplayStyle=1  fundamental=50  FreqAxis=off  MaxFrequency=1000  frequencyindicesteady=1  RmsSteady=1  display=off
  untitledPanel : Subsystem  Tag=HiddenForWebPanel  IsWebBlockPanel=on
  untitledPanel1 : Subsystem  Tag=HiddenForWebPanel  IsWebBlockPanel=on
  wref (pu) : Constant
  tag scope: I_bat=global, PWM=global, gate1=global, gate2=global, genM=global
  wires:
  [duty_B] -> PWM Generator (DC-DC)1/1
  Sum1/1 -> PID Controller1/1
  NOT2/1 -> [gate2]
  Constant3/1 -> Sum1/1
  [v_bus] -> Sum1/2
  [iB_ref] -> Sum/2
  Bus Selector1/2 -> [V_bat]  "<Voltage (V)>"
  Voltage Measurement/1 -> [v_bus]  "V_bus"
  Sum/1 -> PID Controller/1
  Bus Selector1/1 -> [I_bat]  "<Current (A)>"
  PWM Generator (DC-DC)1/1 -> NOT2/1, [gate1]
  Product2/1 -> Mean/1  "P_PV"
  [PWM] -> IGBT/Diode/1
  MPPT/1(Vref) -> Sum9/1
  Relational Operator/1 -> [PWM]
  Repeating Sequence/1 -> Relational Operator/2
  Unit Delay/1 -> Sum9/2, MPPT/1(V)
  Sum9/1 -> PID Controller4/1
  PID Controller4/1 -> Relational Operator/1
  Unit Delay1/1 -> MPPT/2(I)
  Diesel Generator 1MW/1(m) -> [genM]
  Vref (pu)/1 -> Diesel Generator 1MW/2(Vref (pu))
  wref (pu)/1 -> Diesel Generator 1MW/1(wref (pu))
  Bus Selector4/1 -> Gain/1  "<Rotor speed  wm  (pu)>"
  [genM] -> Bus Selector4/1
  [genM] -> Bus Selector3/1
  Repeating Sequence Interpolated2/1 -> Sum3/1, "Total Variable Load "/1(Load)  "Total_Variable_Load"
  Sum3/1 -> Terminator/1  "Total_Load"
  Repeating Sequence Interpolated4/1 -> Terminator1/1, Sum3/2  "Base_Load"
  [P_Gen] -> Scope2/1  "P_Gen"
  Mean/1 -> [P_PV]  "P_PV"
  [P_PV] -> Sum2/1  "Power_Solar"
  [P_Wind] -> Sum2/3  "Power_Wind"
  Sum2/1 -> [PTotal], Divide/2, Subtract/1  "Total_Power"
  [V_bat] -> Product/1  "V_bat"
  [I_bat] -> Product/2  "I_bat"
  Product/1 -> Mean1/1
  [P_bat] -> Sum2/4  "Power_Battery"
  PID Controller1/1 -> Saturation/1
  Saturation/1 -> [iB_ref]  "iB_ref"
  PID Controller/1 -> [duty_B]  "duty_B"
  [I_bat] -> Sum/1
  Wind Turbine 100kW/1(P_Wind) -> [P_Wind]
  User_Irradiance/1 -> Product1/2  "User_Irradiance"
  Excellent_Irradiance/1 -> Multiport Switch/2  "Excellent_Irradiance"
  Typical_Irradiance/1 -> Multiport Switch/3  "Typical_Irradiance"
  Subtract/1 -> Divide/1
  Constant/1 -> Product3/2
  Divide/1 -> Product3/1
  Product3/1 -> Sum4/1, Terminator3/1  "Ren_Penetration"
  Irradiance_Constant/1 -> Product1/1
  Worst_Irradiance/1 -> Multiport Switch/4  "Worst_Irradiance"
  Product1/1 -> Multiport Switch1/3
  Gain/1 -> [freq_following]
  Typical_Power/1 -> Multiport Switch2/3  "Typical_Wind_PG"
  Multiport Switch2/1 -> Multiport Switch3/2
  Product4/1 -> Scope9/1, Multiport Switch3/3  "UserWind"
  WindZeroToOne/1 -> Product4/2
  Worst_Power/1 -> Multiport Switch2/4  "Worst_Wind_PG"
  Wind Speed/1 -> Product4/1
  TypeOfCond/1 -> [Conditions]
  [Conditions] -> Multiport Switch/1
  [Conditions] -> Multiport Switch2/1
  Multiport Switch/1 -> Multiport Switch1/2
  Bus Selector/1 -> [VPV]  "<V_PV>"
  [VPV] -> Unit Delay/1
  Bus Selector/2 -> [IPV]  "<I_PV>"
  [IPV] -> Unit Delay1/1
  [VPV] -> Product2/1
  [IPV] -> Product2/2
  [Conditions] -> Multiport Switch4/1
  Multiport Switch4/1 -> DC/AC PV + Batt/1, DC/AC Wind/1
  Grid-Forming Inverter Controller/1(Pulses Forming) -> Multiport Switch4/2
  Grid-Following Inverter Controller/1(Pulses) -> Multiport Switch4/3
  Switch/1 -> Subtract/2, [PGen]  "P_Gen"
  [Conditions] -> Switch/2
  Mean1/1 -> [P_bat]  "P_Bat"
  Switch1/1 -> Scope/1  "Frequency"
  [Conditions] -> Switch1/2
  Excellent_Power/1 -> Multiport Switch2/2  "Excellent_Wind_PG"
  Constant1/1 -> Switch/3
  [P_Gen] -> Switch/1
  [freq_following] -> Switch1/1
  Constant2/1 -> Switch1/3
  Multiport Switch3/1 -> Wind Turbine 100kW/1(w_s)  "Wind Speed[m/s]"
  [P_bat] -> Subsystem1/1(In1)
  Constant4/1 -> Subsystem1/2(In2)
  Subsystem1/1(SOC_test) -> Scope1/1
  [Conditions] -> Three-Phase Breaker/1
  Digital Clock/1 -> MATLAB Function/6(Time)
  [P_PV] -> MATLAB Function/1(P_PV)  "P_PV"
  [PGen] -> Sum2/2  "Power_Diesel"
  [PGen] -> MATLAB Function/2(P_Gen)  "P_Gen"
  [P_bat] -> MATLAB Function/3(P_Bat)  "P_bat"
  [P_Wind] -> MATLAB Function/4(P_Wind)  "P_Wind"
  [PTotal] -> MATLAB Function/5(P_Total)
  Three-Phase V-I Measurement1/1 -> [Vabcwind]  "Vabc_wind"
  [Vabcwind] -> Scope3/1
  Three-Phase V-I Measurement1/2 -> [Iabcwind]  "Iabc_wind"
  [Iabcwind] -> Scope3/2
  Three-Phase V-I Measurement/1 -> [VabcPV]  "Vabc_PV"
  [VabcPV] -> Scope4/1
  Three-Phase V-I Measurement/2 -> [IabcPV]  "Iabc_PV"
  [IabcPV] -> Scope4/2
  [P_PV] -> Scope6/1
  [v_bus] -> Scope7/1
  [P_Wind] -> Scope8/1
  MATLAB Function/2(DieselEnergy) -> [DieselEnergy]
  [DieselEnergy] -> Scope5/1
  MATLAB Function/3(PVEnergy) -> [PVEnergy]
  [PVEnergy] -> Scope5/2
  MATLAB Function/4(WindEnergy) -> [WindEnergy]
  [WindEnergy] -> Scope5/3
  MATLAB Function/5(BatteryEnergy) -> [BatteryEnergy]
  [BatteryEnergy] -> Scope5/4
  Levelized Cost of Energy/1(LCOE_out) -> Terminator4/1  "LCOE"
  MATLAB Function/1(TotalEnergy) -> Subsystem2/1(Total_Energy_Joules)
  Subsystem2/1(Total_Energy [kWh]) -> Terminator5/1
  CO2 Emissions/1(Kg-CO2/kWh) -> Terminator6/1  "Kg-CO2/kWh"
  [DieselEnergy] -> CO2 Emissions/2(Diesel_energy)
  Unit Delay2/1 -> Divide1/1, Sum4/2
  Sum4/1 -> Unit Delay2/1
  Clock/1 -> Divide1/2
  Divide1/1 -> Gain1/1
  "Battery 6MWh "/1 -> Bus Selector1/1
  Multiport Switch1/1 -> "PV Array "/1  "Irradiance [Wh/m^2]"
  "Average Temperature "/1 -> "PV Array "/2  "Avg. Temp [C]"
  "PV Array "/1 -> Bus Selector/1
  [gate2] -> Mosfet1/1
  [gate1] -> Mosfet/1
  Constant5/1 -> Multiport Switch5/2
  [Conditions] -> Multiport Switch5/1
  Gain1/1 -> Multiport Switch5/3
  Multiport Switch5/1 -> Terminator2/1  "Ren_Avg"
  [Conditions] -> CO2 Emissions/1(Condition)
  Bus Selector3/1 -> [P_Gen]  "<Active Power (W)>"
  [Conditions] -> Levelized Cost of Energy/1(Condition)
  TypeOfCond1/1 -> [Real_or_User]
  [Real_or_User] -> Multiport Switch1/1
  [Real_or_User] -> Multiport Switch3/1
  connections:
  Three-Phase Series RLC Branch/RConn1 -- Three-Phase Parallel RLC Branch/LConn1 -- Three-Phase V-I Measurement/LConn1
  Three-Phase Series RLC Branch/RConn2 -- Three-Phase Parallel RLC Branch/LConn2 -- Three-Phase V-I Measurement/LConn2
  Three-Phase Series RLC Branch/RConn3 -- Three-Phase Parallel RLC Branch/LConn3 -- Three-Phase V-I Measurement/LConn3
  Three-Phase Parallel RLC Branch1/LConn1 -- Three-Phase Series RLC Branch1/RConn1 -- Three-Phase V-I Measurement1/LConn1
  Three-Phase Series RLC Branch1/RConn2 -- Three-Phase Parallel RLC Branch1/LConn2 -- Three-Phase V-I Measurement1/LConn2
  Three-Phase Series RLC Branch1/RConn3 -- Three-Phase Parallel RLC Branch1/LConn3 -- Three-Phase V-I Measurement1/LConn3
  Three-Phase Parallel RLC Branch1/RConn3 -- Three-Phase Parallel RLC Branch1/RConn1 -- Three-Phase Parallel RLC Branch1/RConn2 -- Ground1/LConn1
  Three-Phase Series RLC Branch/LConn2 -- DC/AC PV + Batt/LConn2
  DC/DC Wind/RConn2 -- DC/AC Wind/RConn2
  DC/DC Wind/RConn1 -- DC/AC Wind/RConn1
  Three-Phase Series RLC Branch1/LConn2 -- DC/AC Wind/LConn2
  Three-Phase V-I Measurement/RConn3 -- "Total Variable Load "/RConn3 -- Three-Phase V-I Measurement1/RConn3 -- Grid-Forming Inverter Controller/LConn1 -- Grid-Following Inverter Controller/LConn1 -- Three-Phase Breaker/LConn3 -- " "/LConn3
  "Total Variable Load "/RConn2 -- Grid-Following Inverter Controller/LConn2 -- Three-Phase Breaker/LConn2 -- Three-Phase V-I Measurement/RConn2 -- " "/LConn2 -- Grid-Forming Inverter Controller/LConn2 -- Three-Phase V-I Measurement1/RConn2
  " "/LConn1 -- Grid-Forming Inverter Controller/LConn3 -- Three-Phase V-I Measurement1/RConn1 -- "Total Variable Load "/RConn1 -- Grid-Following Inverter Controller/LConn3 -- Three-Phase Breaker/LConn1 -- Three-Phase V-I Measurement/RConn1
  DC/AC PV + Batt/LConn1 -- Three-Phase Series RLC Branch/LConn1
  DC/AC Wind/LConn3 -- Three-Phase Series RLC Branch1/LConn3
  DC/AC PV + Batt/LConn3 -- Three-Phase Series RLC Branch/LConn3
  DC/AC Wind/LConn1 -- Three-Phase Series RLC Branch1/LConn1
  "      R"/RConn1 -- "Battery 6MWh "/LConn2 -- Mosfet1/RConn1 -- Voltage Measurement/LConn2 -- DC/AC PV + Batt/RConn2 -- Series RLC Branch11/RConn1 -- Series RLC Branch1/RConn1 -- Series RLC Branch2/RConn1 -- IGBT/Diode/RConn1 -- Series RLC Branch9/RConn1 -- "PV Array "/RConn2
  L1/LConn1 -- Mosfet/RConn1 -- Mosfet1/LConn1
  Series RLC Branch1/LConn1 -- Mosfet/LConn1 -- "      R"/LConn1 -- Voltage Measurement/LConn1 -- DC/AC PV + Batt/RConn1 -- Series RLC Branch11/LConn1 -- Diode/RConn1 -- Series RLC Branch2/LConn1
  Ground/LConn1 -- Three-Phase Parallel RLC Branch/RConn1 -- Three-Phase Parallel RLC Branch/RConn2 -- Three-Phase Parallel RLC Branch/RConn3
  Series RLC Branch10/LConn1 -- "PV Array "/RConn1 -- Series RLC Branch9/LConn1
  Series RLC Branch10/RConn1 -- IGBT/Diode/LConn1 -- Diode/LConn1
  Three-Phase Breaker/RConn1 -- Diesel Generator 1MW/RConn1
  Three-Phase Breaker/RConn2 -- Diesel Generator 1MW/RConn2
  Three-Phase Breaker/RConn3 -- Diesel Generator 1MW/RConn3
  Wind Turbine 100kW/RConn1 -- DC/DC Wind/LConn1
  Wind Turbine 100kW/RConn2 -- DC/DC Wind/LConn2
  "Battery 6MWh "/LConn1 -- L1/RConn1

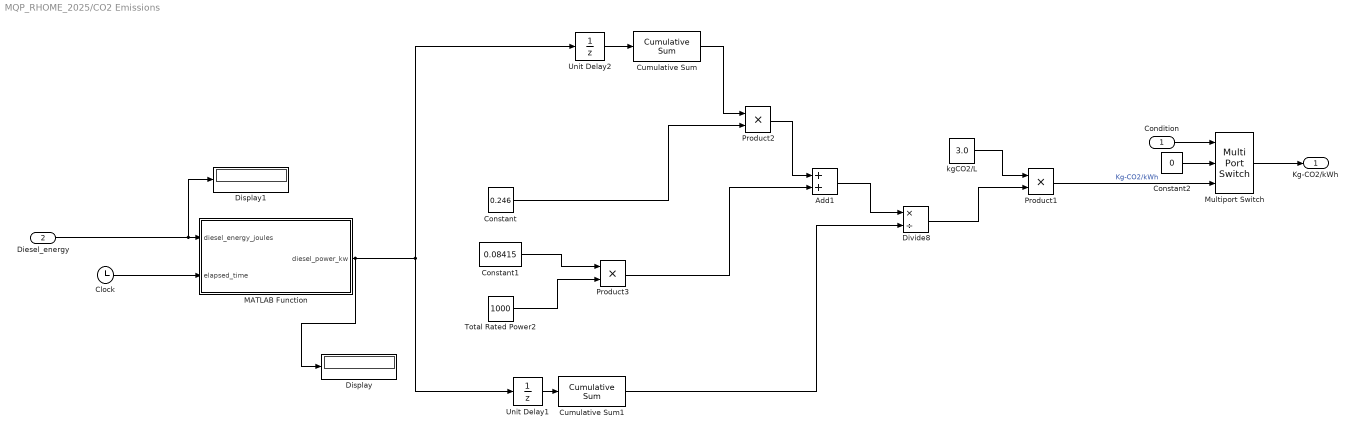
== system MQP_RHOME_2025/CO2 Emissions ==
  Condition : Inport
  Diesel_energy : Inport  Port=2
  Add1 : Sum
  Clock : Clock
  Constant : Constant  Value=0.246
  Constant1 : Constant  Value=0.08415
  Constant2 : Constant  Value=0
  Cumulative Sum : dspmathops/Cumulative Sum  dim=Channels (running sum)  InputProcessing=Columns as channels (frame based)  reset_popup=None  roundingMode=Floor  overflowMode=off  outputDataTypeStr=Inherit: Same as accumulator  outputMin=[]  outputMax=[]  outputLastDataTypeStr=Inherit: Same as accumulator
  Cumulative Sum1 : dspmathops/Cumulative Sum  dim=Channels (running sum)  InputProcessing=Columns as channels (frame based)  reset_popup=None  roundingMode=Floor  overflowMode=off  outputDataTypeStr=Inherit: Same as accumulator  outputMin=[]  outputMax=[]  outputLastDataTypeStr=Inherit: Same as accumulator
  Display : Display
  Display1 : Display
  Divide8 : Product  Inputs=*/
  MATLAB Function : MATLAB Function  TreatAsAtomicUnit=on
  Multiport Switch : MultiPortSwitch  Inputs=2  SaturateOnIntegerOverflow=off  InputSameDT=off
  Product1 : Product
  Product2 : Product
  Product3 : Product
  Total Rated Power2 : Constant  Value=1000
  Unit Delay1 : UnitDelay  HasFrameUpgradeWarning=on
  Unit Delay2 : UnitDelay  HasFrameUpgradeWarning=on
  kgCO2/L : Constant  Value=3.0
  Kg-CO2/kWh : Outport
  wires:
  Divide8/1 -> Product1/2
  Constant/1 -> Product2/2
  Product3/1 -> Add1/2
  kgCO2/L/1 -> Product1/1
  Product2/1 -> Add1/1
  Add1/1 -> Divide8/1
  Total Rated Power2/1 -> Product3/2
  Constant1/1 -> Product3/1
  Unit Delay2/1 -> Cumulative Sum/1
  Cumulative Sum/1 -> Product2/1
  Unit Delay1/1 -> Cumulative Sum1/1
  Cumulative Sum1/1 -> Divide8/2
  Clock/1 -> MATLAB Function/2(elapsed_time)
  MATLAB Function/1(diesel_power_kw) -> Display/1, Unit Delay1/1, Unit Delay2/1
  Condition/1 -> Multiport Switch/1
  Constant2/1 -> Multiport Switch/2
  Product1/1 -> Multiport Switch/3  "Kg-CO2/kWh"
  Multiport Switch/1 -> Kg-CO2/kWh/1
  Diesel_energy/1 -> Display1/1, MATLAB Function/1(diesel_energy_joules)

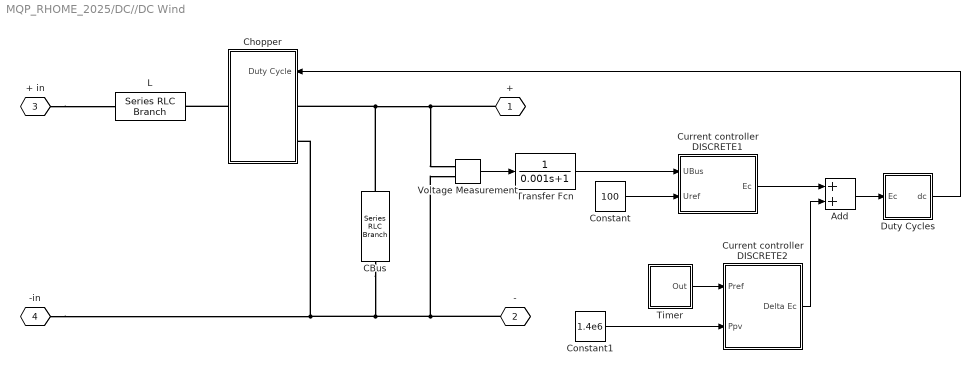
== system MQP_RHOME_2025/DC//DC Wind ==
  Add : Sum
  CBus : spsSeriesRLCBranchLib/Series RLC Branch  LConnTagsString=__new0  RConnTagsString=__new0  BranchType=RC  Resistance=0.2  Inductance=1e-3  SetiL0=off  InitialCurrent=0  Capacitance=7500e-6  Setx0=on  InitialVoltage=100  Measurements=None
  Chopper : Subsystem  mask(SPSdrives Converter){SnubberResistance=10e3, SnubberCapacitance=inf, Ron=1e-3, ForwardVoltages=[1.3,1.3], IGBTParameters=[0,0], converterType=Inverter}
      mask prompts: SnubberResistance "Snubber resistance Rs (Ohms):"; SnubberCapacitance "Snubber capacitance Cs (F):"; Ron "Ron (Ohms):"; ForwardVoltages "Forward voltages [Device Vf(V), Diode Vd (V)]"; IGBTParameters "[Tf(s), Tt(s)]:"; converterType "Converter type:"
      mask help: This model implements an average-value buck converter."Duty Cycle" contains the duty cycle of the internal IGBT device.
      mask TypeOptions converterType: Rectifier | Inverter
      mask Display: plot(0,0,100,100,[39 39 23.8],[71 28 28],[44 56 49.6 56 52.8 56 61 61],[39.2 33.6 32.8 33.6 40.8 33.6 30 12.4],[44 44 44 61 61],[28 71 60 66.4 90],[75 67 83 75 67 83 75 75],[54 42 42 54 54 54 54 66],[61 75 75],[24 24 42],[75 75 61],[66,76,76])
  Constant : Constant  Value=100  SampleTime=1e-6
  Constant1 : Constant  Value=1.4e6
  Current controller DISCRETE1 : Subsystem  mask(PI controller){Kp=0.0005, Ki=0.15, Ts=1e-6}
      mask prompts: Kp "Proportional gain (Kp)"; Ki "Integral gain (Ki)"; Ts "Sample time (s) :"
      mask help: Proportional-Integral Speed Controller
      mask Display: plot(0,0,100,100,[35,35,65],[70,30,30],[35,65],[45,60])
  Current controller DISCRETE2 : Subsystem  mask(PI controller){Kp=0.0005, Ki=0.15, Ts=1e-6}
      mask prompts: Kp "Proportional gain (Kp)"; Ki "Integral gain (Ki)"; Ts "Sample time (s) :"
      mask help: Proportional-Integral Speed Controller
      mask Display: plot(0,0,100,100,[35,35,65],[70,30,30],[35,65],[45,60])
  Duty Cycles : Subsystem
  L : spsSeriesRLCBranchLib/Series RLC Branch  LConnTagsString=__new0  RConnTagsString=__new0  BranchType=L  Resistance=0.3  Inductance=500e-6  SetiL0=off  InitialCurrent=0  Capacitance=100e-6  Setx0=off  InitialVoltage=0  Measurements=None
  Timer : Subsystem  DialogController=POWERSYS.PowerSysDialog  mask(Timer){t=[ 0  1], e=[1 1 ]}
      mask prompts: t "Time (s):"; e "Amplitude:"
      mask help:
      | Generates a signal changing at specified times.
      |
      | If a signal value is not specified at time zero, the output is kept at 0 until the first specified transition time.
      mask init:
      | tt=t;
      | sv=e;
      | if isempty(tt) | isempty(sv)
      | 	% probably during the load process when under a masked block.
      | 	tt=0;
      | 	sv=1;
      | end
      | %
      | if length(sv) ~= length(tt),
      |    Erreur.message = 'The vectors specifying the time and amplitude pairs must have the same length.';
      |    Erreur.identifier = 'SimPowerSystems:TimerBlock:ParameterError';
      |    powericon('psberror',Erreur.message,Erreur.identifier,'NoUiwait');
      | end
      | if tt(1)~=0,
      |    tt=[0 tt];
      |    sv=[~sv(1) sv];
      | end
      | n=length(tt);
      | vec_dt=[tt,0]-[0,tt] ;
      | vec_dt=vec_dt(2:n);
      | if any(vec_dt<=0)
      |    Erreur.message = 'All transition times must be in increasing order.';
      |    Erreur.identifier = 'SimPowerSystems:TimerBlock:ParameterError';
      |    powericon('psberror',Erreur.message,Erreur.identifier,'NoUiwait');
      | end
      | tv=[-1,tt(1),reshape(repmat(reshape(tt(2:end),1,length(tt)-1),2,1),1,2*length(tt)-2),tt(end)+1];
      | %sv=(sv(:)'~=0);
      | opv=[sv(1),reshape(repmat(sv(1:end-1),2,1),1,2*length(sv)-2),sv(end),sv(end)];
      | 
      | power_initmask();
      mask Help: web(psbhelp)
      mask Display: plot( tv(2:end-1), opv(2:end-1) )
  Transfer Fcn : TransferFcn  Denominator=[0.001 1]
  Voltage Measurement : spsVoltageMeasurementLib/Voltage Measurement  PhasorSimulation=off  OutputType=Complex  PSBequivalent=0
  + : PMIOPort  Tag=PMCPort  Side=Right
  - : PMIOPort  Tag=PMCPort  Port=2  Side=Right
  + in : PMIOPort  Tag=PMCPort  Port=3  Side=Left
  -in : PMIOPort  Tag=PMCPort  Port=4  Side=Left
  wires:
  Transfer Fcn/1 -> Current controller DISCRETE1/1(UBus)
  Duty Cycles/1(dc) -> Chopper/1(Duty Cycle)
  Voltage Measurement/1 -> Transfer Fcn/1
  Constant/1 -> Current controller DISCRETE1/2(Uref)
  Timer/1(Out) -> Current controller DISCRETE2/1(Pref)
  Constant1/1 -> Current controller DISCRETE2/2(Ppv)
  Current controller DISCRETE2/1(Delta Ec) -> Add/2
  Add/1 -> Duty Cycles/1(Ec)
  Current controller DISCRETE1/1(Ec) -> Add/1
  connections:
  + in/RConn1 -- L/RConn1
  Chopper/RConn1 -- L/LConn1
  Chopper/LConn2 -- -in/RConn1 -- CBus/RConn1 -- -/RConn1 -- Voltage Measurement/LConn2
  CBus/LConn1 -- Voltage Measurement/LConn1 -- +/RConn1 -- Chopper/LConn1
